simulink model "MARCH_v1_5_stairs"  (R2016a)
settings: Solver=FixedStepDiscrete  StartTime=0.0  StopTime=inf  FixedStep=0.001  RelTol=1e-3
InitFcn:
  | % Change dir to model location
  | cd(fileparts(which(bdroot)));
  | 
  | init_model
  | initialize_model_testingBlocks
StartFcn:
  | cd(fileparts(which(bdroot)));
StopFcn:
  | cd(fileparts(which(bdroot)));
model workspace (MAT data in the model file):
  localValue = 1
  targetValue = 0
undefined symbols (not defined in the file or in its folder): Hip_HAA, Left_Leg, Right_Leg
libraries: xpcethercatlib x71, slrtlib x7, simulink x1, aerolibanimutils x1, dspnetwork x1
(part 2 of 3)

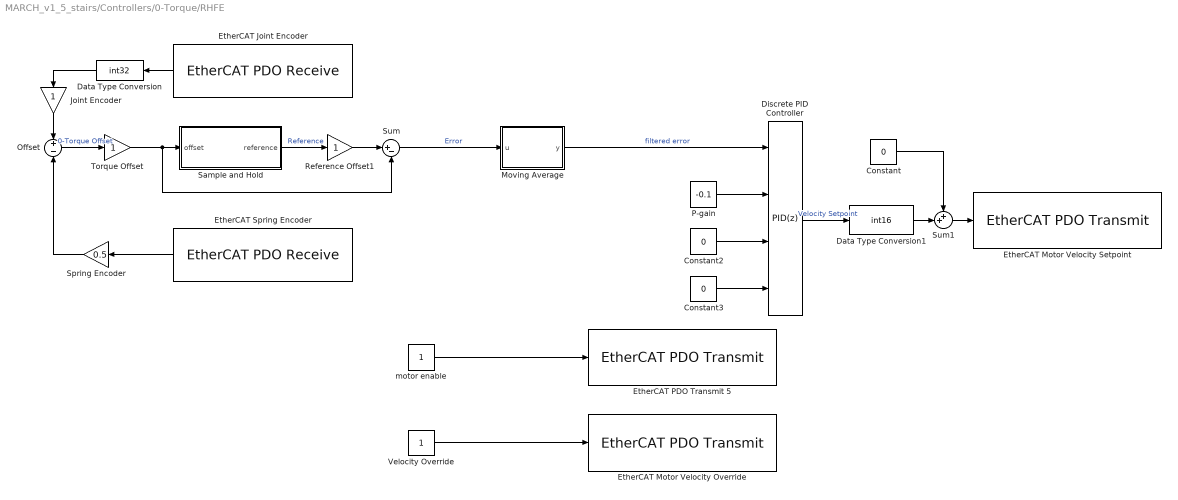
== system MARCH_v1_5_stairs/Controllers/0-Torque/RHFE ==
  Constant : Constant  Value=0  OutDataTypeStr=int16
  Constant2 : Constant  Value=0
  Constant3 : Constant  Value=0
  Data Type Conversion : DataTypeConversion  OutDataTypeStr=int32
  Data Type Conversion1 : DataTypeConversion  OutDataTypeStr=int16
  Discrete PID Controller : simulink/Continuous/PID Controller  Controller=PID  TimeDomain=Discrete-time  SampleTime=-1  IntegratorMethod=Forward Euler  FilterMethod=Forward Euler  Form=Parallel  UseFilter=off  ControllerParametersSource=external  P=-0.7  I=0  D=0  N=100  InitialConditionSource=internal  InitialConditionForIntegrator=0  InitialConditionForFilter=0  ExternalReset=none  LimitOutput=on  UpperSaturationLimit=500  LowerSaturationLimit=-500  LinearizeAsGain=off  AntiWindupMode=none  Kb=1  TrackingMode=off  Kt=1  PParamMin=[]  PParamMax=[]  IParamMin=[]  IParamMax=[]  DParamMin=[]  DParamMax=[]  NParamMin=[]  NParamMax=[]  KbParamMin=[]  KbParamMax=[]  KtParamMin=[]  KtParamMax=[]  POutMin=[]  POutMax=[]  IOutMin=[]  IOutMax=[]  DOutMin=[]  DOutMax=[]  NOutMin=[]  NOutMax=[]  KbOutMin=[]  KbOutMax=[]  KtOutMin=[]  KtOutMax=[]  IntegratorOutMin=[]  IntegratorOutMax=[]  FilterOutMin=[]  FilterOutMax=[]  SumOutMin=[]  SumOutMax=[]  SumOutDataTypeStr=int16  SumI1OutMin=[]  SumI1OutMax=[]  SumI2OutMin=[]  SumI2OutMax=[]  SumI3OutMin=[]  SumI3OutMax=[]  SumDOutMin=[]  SumDOutMax=[]  SaturationOutMin=[]  SaturationOutMax=[]  IntegratorContinuousStateAttributes=''  IntegratorStateMustResolveToSignalObject=off  IntegratorRTWStateStorageClass=Auto  FilterContinuousStateAttributes=''  FilterStateMustResolveToSignalObject=off  FilterRTWStateStorageClass=Auto  DifferentiatorICPrevScaledInput=0  DifferentiatorOutMin=[]  DifferentiatorOutMax=[]
  EtherCAT Joint Encoder : xpcethercatlib/EtherCAT PDO Receive  Priority=2  sig_name=Right_Leg.Inputs.H_jointAngle  sig_offset=1832  sig_type=uint32  type_size=32  sig_dim=1  device_id=0  sample_time=0.001000
  EtherCAT Motor Velocity Override : xpcethercatlib/EtherCAT PDO Transmit   Priority=3  sig_name=Right_Leg.Outputs.H_data[4]  sig_offset=2088  sig_type=int32  type_size=32  sig_dim=1  device_id=0  sample_time=0.001000
  EtherCAT Motor Velocity Setpoint : xpcethercatlib/EtherCAT PDO Transmit   Priority=3  sig_name=Right_Leg.Outputs.H_velocitySetPoint  sig_offset=1832  sig_type=int16  type_size=16  sig_dim=1  device_id=0  sample_time=0.001000
  EtherCAT PDO Transmit 5 : xpcethercatlib/EtherCAT PDO Transmit   Priority=3  sig_name=Right_Leg.Outputs.H_motorEnable  sig_offset=1880  sig_type=uint8  type_size=8  sig_dim=1  device_id=0  sample_time=0.001000
  EtherCAT Spring Encoder : xpcethercatlib/EtherCAT PDO Receive  Priority=2  sig_name=Right_Leg.Inputs.H_springAngle  sig_offset=1864  sig_type=uint32  type_size=32  sig_dim=1  device_id=0  sample_time=0.001000
  Joint Encoder : Gain  OutDataTypeStr=int32
  Moving Average : MATLAB Function  TreatAsAtomicUnit=on
  Offset : Sum  Inputs=+|-
  P-gain : Constant  Value=-0.1
  Reference Offset1 : Gain  OutDataTypeStr=int32
  Sample and Hold : MATLAB Function  TreatAsAtomicUnit=on
  Spring Encoder : Gain  Gain=0.5  OutDataTypeStr=int32
  Sum : Sum  Inputs=|+-  AccumDataTypeStr=uint32
  Sum1 : Sum  Inputs=++|
  Torque Offset : Gain  OutDataTypeStr=int32
  Velocity Override : Constant  OutDataTypeStr=int32
  motor enable : Constant  OutDataTypeStr=uint8
  wires:
  EtherCAT Joint Encoder/1 -> Data Type Conversion/1
  EtherCAT Spring Encoder/1 -> Spring Encoder/1
  Offset/1 -> Torque Offset/1  "0-Torque Offset"
  Sample and Hold/1(reference) -> Reference Offset1/1  "Reference"
  Sum/1 -> Moving Average/1(u)  "Error"
  Velocity Override/1 -> EtherCAT Motor Velocity Override/1
  Spring Encoder/1 -> Offset/2
  Data Type Conversion/1 -> Joint Encoder/1
  Joint Encoder/1 -> Offset/1
  Torque Offset/1 -> Sample and Hold/1(offset), Sum/2
  Reference Offset1/1 -> Sum/1
  Sum1/1 -> EtherCAT Motor Velocity Setpoint/1
  Discrete PID Controller/1 -> Data Type Conversion1/1  "Velocity Setpoint"
  Constant/1 -> Sum1/1
  motor enable/1 -> EtherCAT PDO Transmit 5/1
  Data Type Conversion1/1 -> Sum1/2
  P-gain/1 -> Discrete PID Controller/2
  Constant2/1 -> Discrete PID Controller/3
  Constant3/1 -> Discrete PID Controller/4
  Moving Average/1(y) -> Discrete PID Controller/1  "filtered error"

== system MARCH_v1_5_stairs/Controllers/Continuous Gait/Slider ==

== system MARCH_v1_5_stairs/Controllers/Hold/Motor enable ==
  MotorEnableFlag : Inport
  Demux : Demux  Outputs=6
  Enable LHAA : xpcethercatlib/EtherCAT PDO Transmit   Priority=3  sig_name=Hip_HAA.Outputs.L_motorEnable  sig_offset=256  sig_type=uint8  type_size=8  sig_dim=1  device_id=0  sample_time=0.001000
  Enable LHFE : xpcethercatlib/EtherCAT PDO Transmit   Priority=3  sig_name=Left_Leg.Outputs.H_motorEnable  sig_offset=1192  sig_type=uint8  type_size=8  sig_dim=1  device_id=0  sample_time=0.001000
  Enable LKFE : xpcethercatlib/EtherCAT PDO Transmit   Priority=3  sig_name=Left_Leg.Outputs.K_motorEnable  sig_offset=1480  sig_type=uint8  type_size=8  sig_dim=1  device_id=0  sample_time=0.001000
  Enable RHAA : xpcethercatlib/EtherCAT PDO Transmit   Priority=3  sig_name=Hip_HAA.Outputs.R_motorEnable  sig_offset=560  sig_type=uint8  type_size=8  sig_dim=1  device_id=0  sample_time=0.001000
  Enable RHFE : xpcethercatlib/EtherCAT PDO Transmit   Priority=3  sig_name=Right_Leg.Outputs.H_motorEnable  sig_offset=1880  sig_type=uint8  type_size=8  sig_dim=1  device_id=0  sample_time=0.001000
  Enable RKFE : xpcethercatlib/EtherCAT PDO Transmit   Priority=3  sig_name=Right_Leg.Outputs.K_motorEnable  sig_offset=2168  sig_type=uint8  type_size=8  sig_dim=1  device_id=0  sample_time=0.001000
  wires:
  Demux/3 -> Enable RKFE/1
  Demux/6 -> Enable LKFE/1
  Demux/5 -> Enable LHFE/1
  Demux/2 -> Enable RHFE/1
  MotorEnableFlag/1 -> Demux/1
  Demux/4 -> Enable LHAA/1
  Demux/1 -> Enable RHAA/1

== system MARCH_v1_5_stairs/EtherCAT Joint Setpoints/exoskeleton/EtherCAT Joint Communication ==
  Joint Setpoints : Inport
  Demux : Demux  Outputs=6
  "EtherCAT PDO Transmit " : xpcethercatlib/EtherCAT PDO Transmit   Priority=3  sig_name=Hip_HAA.Outputs.R_jointSetPoint  sig_offset=528  sig_type=uint32  type_size=32  sig_dim=1  device_id=0  sample_time=0.001000
  EtherCAT PDO Transmit 1 : xpcethercatlib/EtherCAT PDO Transmit   Priority=3  sig_name=Right_Leg.Outputs.H_jointSetPoint  sig_offset=1848  sig_type=uint32  type_size=32  sig_dim=1  device_id=0  sample_time=0.001000
  EtherCAT PDO Transmit 2 : xpcethercatlib/EtherCAT PDO Transmit   Priority=3  sig_name=Right_Leg.Outputs.K_jointSetPoint  sig_offset=2136  sig_type=uint32  type_size=32  sig_dim=1  device_id=0  sample_time=0.001000
  EtherCAT PDO Transmit 3 : xpcethercatlib/EtherCAT PDO Transmit   Priority=3  sig_name=Hip_HAA.Outputs.L_jointSetPoint  sig_offset=224  sig_type=uint32  type_size=32  sig_dim=1  device_id=0  sample_time=0.001000
  EtherCAT PDO Transmit 4 : xpcethercatlib/EtherCAT PDO Transmit   Priority=3  sig_name=Left_Leg.Outputs.H_jointSetPoint  sig_offset=1160  sig_type=uint32  type_size=32  sig_dim=1  device_id=0  sample_time=0.001000
  EtherCAT PDO Transmit 5 : xpcethercatlib/EtherCAT PDO Transmit   Priority=3  sig_name=Left_Leg.Outputs.K_jointSetPoint  sig_offset=1448  sig_type=uint32  type_size=32  sig_dim=1  device_id=0  sample_time=0.001000
  wires:
  Demux/5 -> EtherCAT PDO Transmit 4/1
  Demux/6 -> EtherCAT PDO Transmit 5/1
  Demux/4 -> EtherCAT PDO Transmit 3/1
  Demux/1 -> "EtherCAT PDO Transmit "/1
  Demux/2 -> EtherCAT PDO Transmit 1/1
  Joint Setpoints/1 -> Demux/1
  Demux/3 -> EtherCAT PDO Transmit 2/1

== system MARCH_v1_5_stairs/Input Device/Generate random block signal safety/Create peak1 ==
  In1 : Inport
  Delay : Delay  DelayLength=1
  Greater than 0 : MATLAB Function  TreatAsAtomicUnit=on
  Sum : Sum  Inputs=|-+
  Out1 : Outport
  wires:
  Sum/1 -> Greater than 0/1(peak)
  In1/1 -> Sum/2, Delay/1
  Delay/1 -> Sum/1
  Greater than 0/1(signal) -> Out1/1

== system MARCH_v1_5_stairs/Input Device/Generate random block signal safety/Create peak2 ==
  In1 : Inport
  Delay : Delay  DelayLength=1
  Greater than 0 : MATLAB Function  TreatAsAtomicUnit=on
  Sum : Sum  Inputs=|-+
  Out1 : Outport
  wires:
  Sum/1 -> Greater than 0/1(peak)
  In1/1 -> Sum/2, Delay/1
  Delay/1 -> Sum/1
  Greater than 0/1(signal) -> Out1/1

== system MARCH_v1_5_stairs/Input Device/Generate random block signal safety/Create peak3 ==
  In1 : Inport
  Delay : Delay  DelayLength=1
  Greater than 0 : MATLAB Function  TreatAsAtomicUnit=on
  Sum : Sum  Inputs=|-+
  Out1 : Outport
  wires:
  Sum/1 -> Greater than 0/1(peak)
  In1/1 -> Sum/2, Delay/1
  Delay/1 -> Sum/1
  Greater than 0/1(signal) -> Out1/1

== system MARCH_v1_5_stairs/Input Device/Generate random block signal trigger/Create peak1 ==
  In1 : Inport
  Delay : Delay  DelayLength=1
  Greater than 0 : MATLAB Function  TreatAsAtomicUnit=on
  Sum : Sum  Inputs=|-+
  Out1 : Outport
  wires:
  Sum/1 -> Greater than 0/1(peak)
  In1/1 -> Sum/2, Delay/1
  Delay/1 -> Sum/1
  Greater than 0/1(signal) -> Out1/1

== system MARCH_v1_5_stairs/Input Device/Generate random block signal trigger/Create peak2 ==
  In1 : Inport
  Delay : Delay  DelayLength=1
  Greater than 0 : MATLAB Function  TreatAsAtomicUnit=on
  Sum : Sum  Inputs=|-+
  Out1 : Outport
  wires:
  Sum/1 -> Greater than 0/1(peak)
  In1/1 -> Sum/2, Delay/1
  Delay/1 -> Sum/1
  Greater than 0/1(signal) -> Out1/1

== system MARCH_v1_5_stairs/Input Device/Generate random block signal trigger/Create peak3 ==
  In1 : Inport
  Delay : Delay  DelayLength=1
  Greater than 0 : MATLAB Function  TreatAsAtomicUnit=on
  Sum : Sum  Inputs=|-+
  Out1 : Outport
  wires:
  Sum/1 -> Greater than 0/1(peak)
  In1/1 -> Sum/2, Delay/1
  Delay/1 -> Sum/1
  Greater than 0/1(signal) -> Out1/1

== matlab function MARCH_v1_5_stairs/Reachability/MATLAB Function ==
  data: q input size=6; q_out output size=6; err output size=6
function [q_out, err] = fcn(q)

joint_limit_min = [-20 -109 -3 -23 -109 -3]'/180*pi;
joint_limit_max = [23 21 121 20 21 121]'/180*pi;

n = size(q,2);
%% Check if all joints are within limits

err = imag(q)~=0 | q<repmat(joint_limit_min,n,1) | q>repmat(joint_limit_max,n,1);
q_out = q;

== matlab function MARCH_v1_5_stairs/Controllers/Continuous Gait/Trajectory ==
  data: stepHeight input; q output; done output; stepLength input; q input size=[1 6]; torso_z output; debugIn input; base output; debug output
function [q,done, torso_z, base, debug]= fcn(stepHeight,stepLength,q,debugIn)
%#codegen

persistent r splineCtrl i trajectory fullStep fullWeightShift torsoTrajectory weightShiftRatio;

%% Initialize all variables
if(isempty(splineCtrl))
    splineCtrl = splineController();
end

if(isempty(fullStep))
    fullStep = 0;
    fullWeightShift = 0;
end

if(isempty(r))
    % Get frequency of the model
    r = robotics();
    r.base = 1;
    
end

if(isempty(i))
    i = 0;
end

if(isempty(trajectory))
    trajectory = [];
    torsoTrajectory = [];
end

if(isempty(weightShiftRatio))
    weightShiftRatio = 0;
end
%% Logic
% Only run this for the beginning of the swing
r.setTorsoHeight(debugIn);
if(~i)
    
    splineCtrl.method('circle');
    % We set the method of whether we want an analytically generated spline
    % or a spline directly from the database.
    % Options: 'circle' and 'stairs'
    splineCtrl.setStepLength(stepLength).setStepHeight(stepHeight);
    if(~fullStep)
        trajectory = splineCtrl.method('circle').setVelocity(0.7).getHalfStep();
        fullStep = 1;
    else
        trajectory = splineCtrl.method('circle').setVelocity(0.7).getFullStep();
    end
    
    % Transform the spline to the correct frame based on which foot is
    % swinging
    trajectory = r.transformSpline(trajectory);
    
    
    torso_delta = [0 0.0 0];
    
    % Weight shift to base foot
    if(r.base == 1)
        torso_delta(2) = abs(torso_delta(2));
    else
        torso_delta(2) = -abs(torso_delta(2));
    end
    
    if(~fullWeightShift)
        torsoTrajectory = splineCtrl.getHalfWeightShift(torso_delta);
        fullWeightShift = 1;
    else
        torsoTrajectory = splineCtrl.getFullWeightShift(torso_delta);
    end
    
    i = i+1;
end

r.point = [trajectory(1,i) trajectory(2,i) trajectory(3,i)];
debug = r.point;
% r.step(weightShiftRatio(i));
r.weightShift(torsoTrajectory(i,:));

r.inverseKinematics();
q = r.q;

torso_z = r.torso_z;

% Set final values as initial values for the next iteration
r.refresh();

% Reset iterator after we're done with the trajectory, otherwise we
% increment the counter and continue iterating as simulink continues
% sampling
if( i < (length(trajectory)))
    i = i+1;
    done = 0;
else
    i = 0;
    r.switchFoot(r.base);
    done = 1;
end

% Output which foot is currently ON THE GROUND
base = r.base;
end

== matlab function MARCH_v1_5_stairs/Controllers/Continuous Gait/Torso Trajectory ==
  data: desired input; current input; z output
function z = fcn(desired, current)
%#codegen

persistent trajectory i desiredPersistent;

% Speed at which we home in SAMPLES
samples = 1000;

if (isempty(i))
    i = 0;
    
    % Hack to fix initial condition of delay during init phase
    current = desired;
end

if(isempty(desiredPersistent))
    desiredPersistent = desired;
end

if(isempty(trajectory))
    trajectory = linspace(current,desiredPersistent,samples);
end

if(desiredPersistent ~= desired)
    trajectory = linspace(current,desired,samples);
    desiredPersistent = desired;
    i = 0;
end

if(i < samples)
    i = i+1;
end

z = trajectory(i);

== matlab function MARCH_v1_5_stairs/Controllers/Switcher ==
  data: index output; i input; enable output
function [index, enable]= fcn(i)
%#codegen

% This function is supposed to take a state and switch between controllers.
% Currently it directly routes the input argument as the index. In the
% future this can be something different so I have left it open for
% future modifications.

% The u vector represents the controllers. When the vector consists out of
% zeros it will not enable any controller. In the case that an index is set
% to a non zero value, the controller which belongs to that index will be
% enabled.
u = zeros(10,1);

u(i) = 2;

index = i;
enable = u;

== matlab function MARCH_v1_5_stairs/EtherCAT Joint Data In/MATLAB Function ==
  data: encoderValue input; angles output; par parameter
function angles = convertToJointAngles(encoderValue, par)
angles = zeros(6,1);

for i = 1:6
    angles(i) = enc2rad(encoderValue(i), i, par);
end

== matlab function MARCH_v1_5_stairs/Controllers/0-Torque/RHFE/Moving Average ==
  data: u input; y output
function y = fcn(u)

persistent array i;

if(isempty(array))
   array = zeros(1,100);
   i = 1;
end

if(i > 100)
   i = 1; 
end

array(i) = u;
i = i+1;
y = mean(array);

== matlab function MARCH_v1_5_stairs/Controllers/Walking/Trajectory ==
  data: base input; q output; done output; action input; stepType input; q input size=[1 6]; torsoHeight input; stepHeight input; stepLength input; stepVelocity input
function [q,done]= fcn(base,action,stepType, q, torsoHeight,stepHeight, stepLength, stepVelocity)
%#codegen

persistent r splineCtrl i triggerPersistent trajectory hold fullWeightShift timeCurve weightShiftRatio;

%% Initialize all variables
if(isempty(splineCtrl))
    splineCtrl = splineController();
end

if(isempty(fullWeightShift))
    fullWeightShift = 0;
end

% stepType can be 0,1 or 2. 0 = half step forward, 1 is full step, 2 is
% half step trailing
if(isempty(stepType))
    stepType = 0;
end

if(isempty(r))
    % Get frequency of the model
    r = robotics();
    r.base = base;
    timeCurve = [0 0 0];
end

if(isempty(hold))
    hold = 0;
end

if(isempty(i))
    i = 0;
end

if(isempty(triggerPersistent))
    triggerPersistent = action;
end


if(isempty(trajectory))
    trajectory = [0 0 0];
end

if(isempty(weightShiftRatio))
    weightShiftRatio = 0;
end
    
%% Logic
% Only run this for the beginning of the swing
done = 0;

% Reset values if trigger is toggled.
if(triggerPersistent ~= action)
    r.base = base;
    i = 0;
    hold = 0;
    triggerPersistent = action;
end

% Hold exoskeleton in same position after a single step
if(hold)
    q = r.q;
    done = 1;
    return
end

if(~i)
    % weightShiftRatio(end)
    % Foot Trajectory
    splineCtrl.method('circle');
    splineCtrl.setStepHeight(stepHeight).setStepLength(stepLength);
    if(~stepType || stepType == 2)
        trajectory = splineCtrl.method('circle').setVelocity(stepVelocity).getHalfStep();
    else
        trajectory = splineCtrl.method('circle').setVelocity(stepVelocity).getFullStep();
    end
    
    trajectory = r.transformSpline(trajectory);
    
    if(~stepType && r.base == 1)
        weightShiftRatio = linspace(0.5,0.7,length(trajectory));
    end
    
    if(~stepType && r.base == 3)
        weightShiftRatio = linspace(0.5,0.3,length(trajectory));
    end    
    
    % Get trajectory of torso based on the weight shift. WeightShiftRatio
    % is zero --> torso on right foot, WeightShiftRatio is 1 --> torso on
    % left foot
    if(stepType == 1 && r.base == 1)
        weightShiftRatio = linspace(0.3,0.7,length(trajectory));
    end
    
    if(stepType == 1 && r.base == 3)
        weightShiftRatio = linspace(0.7,0.3,length(trajectory));
    end
    
    % Get trajectory of torso based on the weight shift. WeightShiftRatio
    % is zero --> torso on right foot, WeightShiftRatio is 1 --> torso on
    % left foot
    if(stepType == 2 && r.base == 1)
        weightShiftRatio = linspace(0.3,0.5,length(trajectory));
    end
    
    if(stepType == 2 && r.base == 3)
        weightShiftRatio = linspace(0.7,0.5,length(trajectory));
    end

    timeCurve = splineCtrl.getEaseTimeCurve();
    
    i = i+1;
end
r.torso_z = torsoHeight;

r.point = [splineCtrl.easeTrajectory(trajectory(1,:),i,timeCurve) splineCtrl.easeTrajectory(trajectory(2,:),i,timeCurve) splineCtrl.easeTrajectory(trajectory(3,:),i,timeCurve)];
% r.step(); 
r.step(weightShiftRatio(i));
% r.weightShift(torsoTrajectory(i,:));
r.inverseKinematics();

q = r.q;
% torso(i,:) = r.torso;

% Set final values as initial values for the next iteration
r.refresh();

% Reset iterator after we're done with the trajectory, otherwise we
% increment the counter and continue iterating as simulink continues
% sampling
if( i < (length(trajectory)))
    i = i+1;
else
    hold = 1;
end

end

== matlab function MARCH_v1_5_stairs/Controllers/Hold/MATLAB Function ==
  data: q_in input size=[1 6]; action input; q_out output double size=[1 6]; reset input; motorEnable output
function [q_out, motorEnable] = fcn(q_in,action,reset)
persistent q_hold hold action_persistent

if(isempty(q_hold))
   q_hold = zeros(1,6); 
   hold = 0;
end

if (isempty(action_persistent))
    action_persistent = action;
end

if(reset)
   hold = 0; 
end

if (action_persistent ~= action)
    hold = 0;
    action_persistent = action;
end

if(~hold)
    q_hold = q_in;
    hold = 1;
end

motorEnable = uint8(zeros(1,6));

if (hold)
    motorEnable = uint8(ones(1,6));
end

q_out = q_hold;

== matlab function MARCH_v1_5_stairs/Input Device/Generate random block signal safety/Create peak1/Greater than 0 ==
  data: peak input; signal output
function signal  = fcn(peak)


if peak >= 0
    signal = peak;
else
    signal = 0;
    
    
end

== matlab function MARCH_v1_5_stairs/State Machine/Create peak3/Greater than 0 ==
  data: peak input; signal output
function signal  = fcn(peak)


if peak >= 0
    signal = peak;
else
    signal = 0;
    
    
end

== matlab function MARCH_v1_5_stairs/Controllers/Point & Go/Trajectory ==
  data: base input; q output; action input; point input; q input size=[1 6]; debugOut output; debugIn input
function [q,debugOut]= fcn(base,action, point,q,debugIn)
%#codegen

persistent r splineCtrl i triggerPersistent trajectory fullStep hold pointPersistent;

%% Initialize all variables
if(isempty(splineCtrl))
    splineCtrl = splineController();
end


if(isempty(fullStep))
    fullStep = 0;
end

if(isempty(r))
    r = robotics();
    r.base = base;
    
end

if(isempty(hold))
    hold = 0;
end

if(isempty(i))
    i = 0;
end

if(isempty(triggerPersistent))
    triggerPersistent = action;
end

if(isempty(pointPersistent))
    pointPersistent = point;
end

if(isempty(trajectory))
    trajectory = [0 0];
end

%% Logic

% Reset values if trigger is toggled.
if(triggerPersistent ~= action)
    r.base = base;
    i = 0;
    hold = 0;
    triggerPersistent = action;
end


% Hold exoskeleton in same position after a single step
if(hold)
    debugOut = r.torso_z;
    q = r.q;
    return
end

if(~i)
    
    % We set the method of whether we want an analytically generated spline
    % or a spline directly from the database.
    % Options: 'circle' and 'stairs'
    splineCtrl.setStepHeight(0.3);
    trajectory = splineCtrl.method('circle').getStepFromPoint(point);
    
    
    
    % Transform the spline to the correct frame based on which foot is
    % swinging
    trajectory = r.transformSpline(trajectory);
    
    i = i+1;
end

r.point = [trajectory(1,i) trajectory(2,i) trajectory(3,i)];

r.stepPosture();
r.inverseKinematics();

q = r.q;
debugOut = r.torso_z;

% Set final values as initial values for the next iteration
r.refresh();

% Reset iterator after we're done with the trajectory, otherwise we
% increment the counter and continue iterating as simulink continues
% sampling
if( i < (length(trajectory)))
    i = i+1;
else
    hold = 1;
end

end

== matlab function MARCH_v1_5_stairs/State Machine/Input Interpreter Safety ==
  data: rightIn input; rightOut output; leftIn input; leftOut output; bothOut output
function [rightOut, leftOut, bothOut]= fcn(rightIn, leftIn)

persistent countRight countLeft countBoth

if (isempty(countRight)||isempty(countLeft)||isempty(countBoth));
    countRight = 0;
    countLeft = 0;
    countBoth = 0;
    rightOut = 0;
    leftOut = 0;
    bothOut = 0;
end

threshold = 700;


if (rightIn == 0 && leftIn == 0)
    rightOut = 0;
    leftOut = 0;
    bothOut = 0;
    countRight = 0;
    countLeft = 0;
    countBoth = 0;
elseif (rightIn == 1 && leftIn ~= 1)
    countRight = countRight + 1;
    countLeft = 0;
    countBoth = 0;
    if countRight == threshold
        rightOut = 1;
        leftOut = 0;
        bothOut = 0;
        countRight = 0;
    else
        rightOut = 0;
        leftOut = 0;
        bothOut = 0;
    end
elseif (leftIn == 1 && rightIn ~= 1)
    countRight = 0;
    countLeft = countLeft + 1;
    countBoth = 0;
    if countLeft == threshold
        rightOut = 0;
        leftOut = 1;
        bothOut = 0;
        countLeft = 0;
    else
        rightOut = 0;
        leftOut = 0;
        bothOut = 0;
    end
elseif (rightIn == 1 && leftIn == 1)
    countRight = 0;
    countLeft = 0;
    countBoth = countBoth + 1;
    if countBoth == threshold
        rightOut = 0;
        leftOut = 0;
        bothOut = 1;
    else
        rightOut = 0;
        leftOut = 0;
        bothOut = 0;
    end
else
    rightOut = -1;
    leftOut = -1;
    bothOut = -1;
end

== matlab function MARCH_v1_5_stairs/EtherCAT Joint Setpoints/exoskeleton/MATLAB Function ==
  data: jointAngle input; encVal output; par parameter
function encVal = convertToEncoderValues(jointAngle, par)
encVal = zeros(6,1);

for i = 1:6
    encVal(i) = rad2enc(jointAngle(i), i, par);
end

== matlab function MARCH_v1_5_stairs/Controllers/StandUp/Trajectory ==
  data: done output; q output; action input; q_i input size=[1 6]; debugIn input
function [done,q] = fcn(action,q_i,debugIn)
%#codegen

persistent r splineCtrl i q_t n hipDelay;

%% Initialize all variables
if(isempty(splineCtrl))
    splineCtrl = splineController();
end

if(isempty(r))
    % Get frequency of the model
    r = robotics();
    
end

if(isempty(q_t))
    q_t = [0 0 0 0 0 0];
    hipDelay = [0 0];
end

if(isempty(i))
    i = 0;
    n = 0;
end


%% Logic
done = 0;

% Prepare for standup by moving the hip forward
if(n == 0 && i == 0)
    q_f = [0 -1.9 q_i(3) 0 -1.9 q_i(6)];
    splineCtrl.samples = 1500;
    q_t = splineCtrl.getJointTrajectory(q_i,q_f);
   
    i = i+1;
end

% Run startup procedure
if(n == 1 && i == 0)
    % Calculate final position based on robotics parameters
    r.setTorsoHeight(debugIn);
    r.refresh();
    r.inverseKinematics();
    q_f = r.q;
    
    splineCtrl.samples = 3000;
    q_t = splineCtrl.getJointTrajectory(q_i,q_f);

    % The hip rotation will play back halfway through the samples
    hipDelay = splineCtrl.getCustomEaseTimeCurve(0.3,1);
    
    i = i+1;
    %q_t = splineCtrl.ease(q_t);
end

q = q_t(i,:);

% Slow down the hip trajectory only when standing up
if(n == 1)
    q(2) = splineCtrl.easeTrajectory(q_t(:,2),i,hipDelay);
    q(5) = splineCtrl.easeTrajectory(q_t(:,5),i,hipDelay);
end

if(i < length(q_t))
    i = i+1;
else
    if(n == 0)
        % Reset iterator
        i = 0;
        n = 1;
    else
        done = 1;
    end
end

end

== matlab function MARCH_v1_5_stairs/State Machine/Input Interpreter Triggers ==
  data: rightIn input; rightOut output; leftIn input; leftOut output; bothOut output
function [rightOut, leftOut, bothOut]= fcn(rightIn, leftIn)

persistent countRight countLeft countBoth

if (isempty(countRight)||isempty(countLeft)||isempty(countBoth));
    countRight = 0;
    countLeft = 0;
    countBoth = 0;
    rightOut = 0;
    leftOut = 0;
    bothOut = 0;
end

threshold = 700;


if (rightIn == 0 && leftIn == 0)
    rightOut = 0;
    leftOut = 0;
    bothOut = 0;
    countRight = 0;
    countLeft = 0;
    countBoth = 0;
elseif (rightIn == 1 && leftIn ~= 1)
    countRight = countRight + 1;
    countLeft = 0;
    countBoth = 0;
    if countRight == threshold
        rightOut = 1;
        leftOut = 0;
        bothOut = 0;
        countRight = 0;
    else
        rightOut = 0;
        leftOut = 0;
        bothOut = 0;
    end
elseif (leftIn == 1 && rightIn ~= 1)
    countRight = 0;
    countLeft = countLeft + 1;
    countBoth = 0;
    if countLeft == threshold
        rightOut = 0;
        leftOut = 1;
        bothOut = 0;
        countLeft = 0;
    else
        rightOut = 0;
        leftOut = 0;
        bothOut = 0;
    end
elseif (rightIn == 1 && leftIn == 1)
    countRight = 0;
    countLeft = 0;
    countBoth = countBoth + 1;
    if countBoth == threshold
        rightOut = 0;
        leftOut = 0;
        bothOut = 1;
    else
        rightOut = 0;
        leftOut = 0;
        bothOut = 0;
    end
else
    rightOut = -1;
    leftOut = -1;
    bothOut = -1;
end

== matlab function MARCH_v1_5_stairs/Controllers/Stairs/Torso Trajectory ==
  data: desired input; torsoTrajectory output size=[1 3]
function torsoTrajectory = fcn(desired)
%#codegen

persistent trajectory i desiredPersistent;

% Speed at which we home in SAMPLES
samples = 1000;

if (isempty(i))
    i = 0;
end

if(isempty(desiredPersistent))
    desiredPersistent = desired;
end

if(isempty(trajectory))   
    desiredPersistent = desired;
    
    trajectory = [linspace(0,desiredPersistent(1),samples)
        linspace(0,desiredPersistent(2),samples)
        linspace(0,desiredPersistent(3),samples) ]';
end

if(~isequal(desiredPersistent,desired))
    trajectory = [linspace(0,desired(1),samples)
        linspace(0,desired(2),samples)
        linspace(0,desired(3),samples) ]';
    
    desiredPersistent = desired;
    i = 0;
end

if(i < samples)
    i = i+1;
end

torsoTrajectory = trajectory(i,:);

== matlab function MARCH_v1_5_stairs/Controllers/Stairs/Trajectory ==
  data: base input; q output; action input; q input size=[1 6]; stepVelocity input; stepLength input; stairHeight input; seq input; done output
function [q,done] = fcn(base,action,q,stepVelocity,stepLength,stairHeight,seq)
%#codegen

persistent r s i j k l m hold trajectory weightShiftRatio timeCurve splineCtrl triggerPersistent;

%% Initialize all variables
if(isempty(splineCtrl))
    splineCtrl = splineController();
end

if(isempty(r))
    % Get frequency of the model
    r = robotics();
    r.base = base;
end

if(isempty(i) || isempty(j) || isempty(k) || isempty(l))
    i = 0;
    j = 0;
    k = 0;
    l = 0;
    m = 0;
end

if(isempty(trajectory))
    trajectory = [0 0 0];
end

if(isempty(triggerPersistent))
    triggerPersistent = action;
end

if(isempty(weightShiftRatio))
    weightShiftRatio = 0;
end

if(isempty(timeCurve))
    timeCurve = 0;
end

if(isempty(hold))
    hold = 0;
end

%% Logic
done = 0;

% Reset values if trigger is toggled.
if(triggerPersistent ~= action)
    r.base = base;
    i = 0;
    hold = 0;
    triggerPersistent = action;
end

% Hold exoskeleton in same position after a single step
if(hold)
    q = r.q;
    done = 1;
    return
end

% Initialisation of number of samples by use of the step Length and the
% step Velocity
splineCtrl.setStepLength(stepLength).setVelocity(stepVelocity).setStairHeight(stairHeight);
%% Weight shifting sequence
% This sequence will weight shift to the base leg. The entire sequence is
% wrapped inside an if statement to prevent this from executing after it
% has been completed. It is either this or a separate function block which
% would be a disaster because the classes are separate instances.


if(seq == 1)
    if (~i)
        r.torso_z = 0.9499;
        r.refresh(); % make sure initial position of torso has same heighit as set above
        
       % I tried to make a smooth weightShift using easeTrajectory but was
       % unsuccessfull, this is far out the fastest and easist solution.
        weightShiftRatio = splineCtrl.getWeightShiftRatioSpacing(0.5, 0.3);  
        
        i = i + 1;      
    end
    
    % Playback trajectory and return preventing doing the rest
    if(i < length(weightShiftRatio))
        r.weightShift(weightShiftRatio(i));
        r.inverseKinematics();
        q = r.q;
        i = i + 1;
    else
        q = r.q;
        
        % Init and enable step sequence
        r.refresh();
        j = 0; 
        done = 1;
        hold = 1;
    end
end

%% Step Sequence
% This sequence will step onto the stair
if(seq == 2)
    if(~j)
        r.base = base;
        % Generate the trajectory based on specific velocity (in m/s) for putting
        % the first leg on the stairs step
        trajectory = splineCtrl.method('stairs_lift').setStepLength(stepLength).setVelocity(stepVelocity).setStepHeightStairs().getStairStep();
        
        % Transform spline to location of foot
        trajectory = r.transformSpline(trajectory);
        
        % Perform the weightShift
        weightShiftRatio = linspace(weightShiftRatio(end),weightShiftRatio(end),length(trajectory));
        timeCurve = splineCtrl.getEaseTimeCurve();
        j = j + 1;
    end
    
    r.point = [splineCtrl.easeTrajectory(trajectory(1,:),j,timeCurve) splineCtrl.easeTrajectory(trajectory(2,:),j,timeCurve) splineCtrl.easeTrajectory(trajectory(3,:),j,timeCurve)];
    r.step(weightShiftRatio(j));
    r.inverseKinematics();
    q = r.q;

    r.refresh();
    
    if(j < length(trajectory))
        j = j+1;
    else
        j = 0;
        q = r.q;
        hold = 1;
        done = 1;
    end
    
end

%% Weightshift on stairs
% This sequence will make the weight be shifted on the leg on the stair
if(seq == 3)
    if(~k)
        r.base = base;
        % I tried to make a smooth weightShift using easeTrajectory but was
        % unsuccessfull, this is far out the fastest and easist solution.
        weightShiftRatio = splineCtrl.getWeightShiftRatioSpacing(weightShiftRatio(end), 0.7);
        
        k = k + 1;
    end
    
    % Playback trajectory and return preventing doing the rest
   
    r.weightShift(weightShiftRatio(k));
    r.inverseKinematics();
    q = r.q;
    
    r.refresh();
 
    if(k < length(weightShiftRatio))
        k = k + 1;
    else
        k = 0;
        q = r.q;
        
        % Init and enable step sequence
        r.refresh();
        k = 0;
        done = 1;
        hold = 1;
    end
end

%% Lifting the trailing leg
% This sequence will left the other leg on the stairs
if(seq == 4)
    if(~l)
        r.base = base;
        % Generate the trajectory based on specific velocity (in m/s) for putting
        % the first leg on the stairs step
        trajectory = splineCtrl.setStepLength(stepLength).setVelocity(stepVelocity).setStepHeightStairs().getTrailingStairStep();
        
        % Transform spline to location of foot
        trajectory = r.transformSpline(trajectory);
        
        weightShiftRatio = linspace(weightShiftRatio(end),weightShiftRatio(end),length(trajectory));
        
        timeCurve = splineCtrl.getEaseTimeCurve();
        
        l = l + 1;
    end 
    
    r.point = [splineCtrl.easeTrajectory(trajectory(1,:),l,timeCurve) splineCtrl.easeTrajectory(trajectory(2,:),l,timeCurve) splineCtrl.easeTrajectory(trajectory(3,:),l,timeCurve)];
    r.step(weightShiftRatio(l));
    r.inverseKinematics();
    q = r.q;

    r.refresh();
    
    if(l < length(trajectory))
        l = l+1;
    else
        l = 0;
        q = r.q;
        hold = 1;
        done = 1;
    end
    
end

%% Making the weightShift back to the middle
% This sequence shifts the MARCH back to the starting position
if(seq == 5)
    if(~m) 
        r.base = base;
        
        % I tried to make a smooth weightShift using easeTrajectory but was
        % unsuccessfull, this is far out the fastest and easist solution.
        weightShiftRatio = splineCtrl.getWeightShiftRatioSpacing(weightShiftRatio(end), 0.5); 
        
        m = m + 1;
    end
        
    r.weightShift(weightShiftRatio(m));
    r.inverseKinematics();
    q = r.q;
   
    r.refresh();
 
    if(m < length(weightShiftRatio))
        m = m + 1;
    else
        m = 0;
        q = r.q;
        
        % Init and enable step sequence
        r.refresh();
        m = 0;
        done = 1;
        hold = 1;
    end
end

weightShiftRatio(end)
end

== matlab function MARCH_v1_5_stairs/Controllers/0-Torque/RHFE/Sample and Hold ==
  data: offset input; reference output
function reference = fcn(offset)
%#codegen

persistent offsetPersistent hold;

if(isempty(offsetPersistent))
    offsetPersistent = int32(0);
    hold = 0;
end

if(offset > 0 && hold == 0)
    
    offsetPersistent = offset;
    hold = 1;
end

reference = offsetPersistent;

== stateflow chart MARCH_v1_5_stairs/State Machine/State Machine ==
  state InputDeviceCheck [commented out]
    en: controllerIndex = 1;
    en: action = 0;
    en: base = 0;
    en: stepType = 0;
    en: state = 0;
    state checkScrollClick [commented out]
      en: inpDevWorking = 0;
    state checkBothSafety [commented out]
      en: inpDevWorking = 0;
    state checkbothTrigger [commented out]
      en: inpDevWorking = 0;
    state InpDev [commented out]
      en: inpDevWorking = 1;
    (default) -> checkScrollClick [commented out] : [rightScrollMode == 1]
    checkScrollClick -> checkBothSafety [commented out] : [rightScrollClick == 1]
    checkBothSafety -> checkbothTrigger [commented out] : [bothSafety == 1]
    checkbothTrigger -> InpDev [commented out] : [bothTriggers == 1]
  state ZeroTorque
    en: controllerIndex = 1;
    en: action = 0;
    en: base = 0;
    en: stepType = 0;
    en: state = 1;
  state testingBypass
    en: controllerIndex = 1;
    en: action = 0;
    en: base = 0;
    en: stepType = 0;
    en: state = 9;
  state SitDown
    en: controllerIndex = 4;
    en: action = 0;
    en: base = 0;
    en: stepType = 0;
    en: state = 4;
  state HoldPosition
    en: controllerIndex = 2;
    en: action = 0;
    en: base = 0;
    en: stepType = 0;
    en: state = 2;
  state StandUp
    en: controllerIndex = 3;
    en: action = 0;
    en: base = 0;
    en: stepType = 0;
    en: state = 3;
  state HoldPosition1
    en: controllerIndex = 2;
    en: action = 0;
    en: base = 0;
    en: stepType = 0;
    en: state = 2;
  state DiscreteGait
    en: controllerIndex = 5;
    state standbyModeDiscr
      en: action = actionLocal;
      en: base = baseLocal;
      en: stepType = 0;
      en: state = 61;
      % satandby mode from discrete gait
      % exoskeleton finishes full step, makes complementary halfstep, then stands still
    state makeLeftHalfStepDiscr
      en: action = action+1;
      en: base = 1;
      en: stepType = 2;
      en: state = 61;
      baseLocal = base;
      actionLocal = action;
    state makeRightHalfStepDiscr
      en: action = action+1;
      en: base = 3;
      en: stepType = 2;
      en: state = 61;
      baseLocal = base;
      actionLocal = action;
    state startLeftHalfStepDiscr
      en: action = 1;
      en: base = 1;
      en: stepType = 0;
      en: state = 6;
      baseLocal = base
    state finishRightFullStepDiscr
      en: action = actionLocal;
      en: base = 3;
      en: stepType = 1;
      en: state = 61;
      baseLocal = base;
      % exoskeleton finishes right full step
    state finishLeftFullStepDiscr
      en: action = actionLocal;
      en: base = 1;
      en: stepType = 1;
      en: state = 61;
      baseLocal = base;
      % exoskeleton finishes left full step
    state makeLeftHalfStepDiscr1
      en: action = action+1;
      en: base = 1;
      en: stepType = 0;
      en: state = 62;
      baseLocal = base;
      actionLocal = action;
    state makeRightHalfStepDiscr3
      en: action = action+1;
      en: base = 3;
      en: stepType = 0;
      en: state = 62;
      baseLocal = base;
      actionLocal = action;
    state leftFullStepDiscr
      en: action = action+1;
      en: base = 1;
      en: stepType = 1;
      en: state = 6;
      baseLocal = base;
      actionLocal = action;
    state rightFullStepDiscr
      en: action = action+1;
      en: base = 3;
      en: stepType = 1;
      en: state = 6;
      baseLocal = base;
      actionLocal = action;
    state safeDiscr2Walk1
      en: action = actionLocal;
      en: base = baseLocal;
      en: stepType = 1;
      en: state = 62;
    state safeDiscr2Walk
      en: action = actionLocal;
      en: base = baseLocal;
      en: stepType = 1;
      en: state = 62;
    state safeModeDiscr
      en: action = actionLocal;
      en: base = baseLocal;
      en: stepType = 1;
      en: state = 62;
      % safemode from discr. gait
      % exoskeleton finishes full step, then stands still
    makeRightHalfStepDiscr3 -> standbyModeDiscr : [done == 1]
    makeLeftHalfStepDiscr1 -> standbyModeDiscr : [done == 1]
    standbyModeDiscr -> startLeftHalfStepDiscr [order 2] : [bothTriggers == 1]
    makeLeftHalfStepDiscr -> standbyModeDiscr : [done == 1]
    makeRightHalfStepDiscr -> standbyModeDiscr : [done == 1]
    finishLeftFullStepDiscr -> makeRightHalfStepDiscr : [done == 1]
    finishRightFullStepDiscr -> makeLeftHalfStepDiscr : [done == 1]
    startLeftHalfStepDiscr -> rightFullStepDiscr : [done == 1 && rightTrigger == 1]
    leftFullStepDiscr -> finishLeftFullStepDiscr [order 1] : [bothTriggers == 1]
    rightFullStepDiscr -> finishRightFullStepDiscr [order 1] : [bothTriggers == 1]
    (junction 178) -> makeRightHalfStepDiscr3 [order 2] : [baseLocal == 1]
    (junction 178) -> makeLeftHalfStepDiscr1 [order 1] : [baseLocal == 3]
    rightFullStepDiscr -> leftFullStepDiscr [order 2] : [done == 1 && leftTrigger ==  1]
    leftFullStepDiscr -> rightFullStepDiscr [order 2] : [done == 1 && rightTrigger == 1]
    safeDiscr2Walk1 -> leftFullStepDiscr [order 2] : [leftTrigger == 1 && baseLocal == 3]
    leftFullStepDiscr -> safeModeDiscr [order 3] : [bothSafety == 1]
    rightFullStepDiscr -> safeModeDiscr [order 3] : [bothSafety == 1]
    safeDiscr2Walk1 -> rightFullStepDiscr [order 1] : [rightTrigger == 1 && baseLocal == 1]
    safeDiscr2Walk -> safeDiscr2Walk1 : [done == 1]
    safeModeDiscr -> safeDiscr2Walk [order 1] : [bothSafety == 1]
    safeModeDiscr -> (junction 178) [order 2] : [bothTriggers == 1 && done == 1]
  state ContinuousGait
    en: controllerIndex = 5;
    state standbyModeCont
      en: action = actionLocal;
      en: base = baseLocal;
      en: stepType = 0;
      en: state = 51;
      % satandby mode from continuous gait
      % exoskeleton finishes full step, makes complementary halfstep, then stands still
    state makeLeftHalfStepCont
      en: action = action+1
      en: base = 1;
      en: stepType = 0;
      en: state = 51;
      baseLocal = base;
    state makeRightHalfStepCont
      en: action = action+1;
      en: base = 3;
      en: stepType = 0;
      en: state = 51;
      baseLocal = base;
      actionLocal = action;
    state startLeftHalfStepCont
      en: action = 1;
      en: base = 1;
      en: stepType = 0;
      en: state = 5;
      baseLocal = base
    state finishLeftFullStepCont
      en: action = actionLocal;
      en: base = 1;
      en: stepType = 1;
      en: state = 51;
      baseLocal = base;
      % exoskeleton finishes left full step
    state finishRightFullStepCont
      en: action = actionLocal
      en: base = 3;
      en: stepType = 1;
      en: state = 51;
      baseLocal = base;
      % exoskeleton finishes right full step
    state makeRightHalfStepCont1
      en: action = action+1;
      en: base = 3;
      en: stepType = 0;
      en: state = 52;
      baseLocal = base;
      actionLocal = action;
    state makeLeftHalfStepCont1
      en: action = action+1;
      en: base = 1;
      en: stepType = 0;
      en: state = 52;
      baseLocal = base;
      actionLocal = action
    state leftFullStepCont
      en: action = action+1;
      en: base = 1;
      en: stepType = 1;
      en: state = 5;
      baseLocal = base;
      actionLocal = action;
    state rightFullStepCont
      en: action = action+1
      en: base = 3;
      en: stepType = 1;
      en: state = 5;
      baseLocal = base;
      actionLocal = action;
    state safeCont2Walk
      en: action = actionLocal;
      en: base = baseLocal;
      en: stepType = 1;
      en: state = 52;
    state safeModeCont
      en: action = actionLocal;
      en: base = baseLocal;
      en: stepType = 1;
      en: state = 52;
      % safemode from cont. gait
      % exoskeleton finishes full step, then stands still
    makeRightHalfStepCont1 -> standbyModeCont : [done == 1]
    standbyModeCont -> startLeftHalfStepCont [order 2] : [bothTriggers == 1]
    makeLeftHalfStepCont1 -> standbyModeCont : [done == 1]
    makeRightHalfStepCont -> standbyModeCont : [done == 1]
    makeLeftHalfStepCont -> standbyModeCont : [done == 1]
    finishLeftFullStepCont -> makeRightHalfStepCont : [done == 1]
    finishRightFullStepCont -> makeLeftHalfStepCont : [done == 1]
    startLeftHalfStepCont -> rightFullStepCont : [done == 1]
    leftFullStepCont -> finishLeftFullStepCont [order 2] : [bothTriggers == 1]
    rightFullStepCont -> finishRightFullStepCont [order 1] : [bothTriggers == 1]
    (junction 172) -> makeRightHalfStepCont1 [order 2] : [baseLocal == 1]
    (junction 172) -> makeLeftHalfStepCont1 [order 1] : [baseLocal == 3]
    leftFullStepCont -> rightFullStepCont [order 3] : [done == 1]
    rightFullStepCont -> leftFullStepCont [order 3] : [done == 1]
    safeCont2Walk -> rightFullStepCont [order 1] : [done == 1 && baseLocal == 1]
    rightFullStepCont -> safeModeCont [order 2] : [bothSafety == 1]
    leftFullStepCont -> safeModeCont [order 1] : [bothSafety == 1]
    safeCont2Walk -> leftFullStepCont [order 2] : [done == 1 && baseLocal == 3]
    safeModeCont -> safeCont2Walk [order 1] : [bothSafety == 1]
    safeModeCont -> (junction 172) [order 2] : [bothTriggers == 1 && done == 1]
  state StairsWalking
    en: controllerIndex = 8;
    state initialWeightShift
      entry: action = 1;
      en: seq = 1;
      en: base = 1;
    state weightShiftStartingPosition
      en: action = action + 1;
      en: seq = 5;
      en: base = 1;
    state firstStepStairsLeftLeg
      en: action = action + 1;
      en: seq = 2;
      en: base = 1;
    state liftLegStairs
      en: action = action + 1;
      en: seq = 4;
      en: base = 3;
    state weightShiftStair
      en: action = action + 1;
      en: seq = 3;
      en: base = 3;
    initialWeightShift -> firstStepStairsLeftLeg : [done == 1]
    weightShiftStartingPosition -> initialWeightShift [order 1] : [done == 1 && rightScrollClick == 1]
    firstStepStairsLeftLeg -> weightShiftStair : [done == 1]
    liftLegStairs -> weightShiftStartingPosition : [done == 1]
    weightShiftStair -> liftLegStairs : [done == 1]
  (default) -> InputDeviceCheck [commented out] : [rightScrollMode == 0]
  checkScrollClick -> testingBypass [commented out] : [rightScrollMode == 9]
  (default) -> ZeroTorque
  ZeroTorque -> HoldPosition [order 1] : [rightScrollMode == 3 && rightScrollClick == 1]
  SitDown -> ZeroTorque [order 1] : [rightScrollMode == 1 && rightScrollClick == 1 && done == 1]
  HoldPosition -> ZeroTorque [order 1] : [rightScrollMode == 1 && rightScrollClick == 1]
  ZeroTorque -> startLeftHalfStepCont [order 3] : [rightScrollMode == 11]
  ZeroTorque -> initialWeightShift [order 2] : [rightScrollMode == 12]
  testingBypass -> HoldPosition : [rightScrollClick == 1]
  HoldPosition1 -> SitDown [order 1] : [rightScrollMode ==4 && rightScrollClick == 1]
  SitDown -> StandUp [order 2] : [rightScrollMode == 3 && rightScrollClick == 1 && done == 1]
  HoldPosition -> StandUp [order 2] : [rightScrollMode == 3 && bothTriggers == 1]
  StandUp -> HoldPosition1 : [done == 1]
  standbyModeCont -> HoldPosition1 [order 1] : [rightScrollMode == 3 && rightScrollClick == 1]
  standbyModeDiscr -> HoldPosition1 [order 1] : [rightScrollMode == 3 && rightScrollClick == 1]
  weightShiftStartingPosition -> HoldPosition1 [order 2] : [rightScrollMode == 3 && rightScrollClick == 1]
  HoldPosition1 -> startLeftHalfStepCont [order 2] : [rightScrollMode == 5 && rightScrollClick == 1]
  HoldPosition1 -> startLeftHalfStepDiscr [order 3] : [rightScrollMode == 6 && rightScrollClick == 1]
  weightShiftStartingPosition -> startLeftHalfStepDiscr [order 3] : [done ==1 && rightScrollMode == 13]
  data: rightTrigger input; leftTrigger input; bothTriggers input; rightSafety input; leftSafety input; bothSafety input; rightScrollMode input; rightScrollClick input; controllerIndex output; action output; base output; inpDevWorking local; done input; stepType output; state output; baseLocal local; actionLocal local; seq output

== matlab function MARCH_v1_5_stairs/Input Device/Generate random block signal safety/Create peak2/Greater than 0 ==
  data: peak input; signal output
function signal  = fcn(peak)


if peak >= 0
    signal = peak;
else
    signal = 0;
    
    
end

== matlab function MARCH_v1_5_stairs/Input Device/Generate random block signal safety/Create peak3/Greater than 0 ==
  data: peak input; signal output
function signal  = fcn(peak)


if peak >= 0
    signal = peak;
else
    signal = 0;
    
    
end

== matlab function MARCH_v1_5_stairs/Input Device/Generate random block signal safety/Rand. Block Func. Gen.1 ==
  data: u input; delayDurationInp input; blockDurationInp input; output output
function output  = fcn(u, delayDurationInp, blockDurationInp)

%% initialize the variable
persistent delayDuration blockDuration

if(isempty(blockDuration)||isempty(delayDuration))
    blockDuration = 0;
    delayDuration = 0;
    output = 0;
end

%% check if the delay and the block are done

doneDelay = (delayDuration <= 0);
doneBlock = (blockDuration <= 0);
done = (doneDelay && doneBlock);



%% Create delay and Block

if (u == 0 && done)
    output = 0;
elseif u == 1
    delayDuration = floor(1000*delayDurationInp);
    output = 0;
elseif not(doneDelay)
    delayDuration = delayDuration - 1;
    output = 0;
    if delayDuration == 0
        blockDuration = floor(1000*blockDurationInp);
        output = 1;
    end
elseif not(doneBlock)
    blockDuration = blockDuration - 1;
    output = 1;
else
    output = -1;
end


end

== matlab function MARCH_v1_5_stairs/Input Device/Generate random block signal safety/Rand. Block Func. Gen.4 ==
  data: delayDurationInp input; blockDurationInp input; u input; output output
function output  = fcn(delayDurationInp, blockDurationInp, u)

%% initialize the variable
persistent delayDuration blockDuration

if(isempty(blockDuration)||isempty(delayDuration))
    blockDuration = 0;
    delayDuration = 0;
    output = 0;
end



%% check if the delay and the block are done

doneDelay = (delayDuration <= 0);
doneBlock = (blockDuration <= 0);
done = (doneDelay && doneBlock);



%% Create delay and Block

if (u == 0 && done)
    output = 0;
elseif u == 1
    delayDuration = floor(1000*delayDurationInp);
    output = 0;
elseif not(doneDelay)
    delayDuration = delayDuration - 1;
    output = 0;
    if delayDuration == 0
        blockDuration = floor(1000*blockDurationInp);
        output = 1;
    end
elseif not(doneBlock)
    blockDuration = blockDuration - 1;
    output = 1;
else
    output = -1;
end


end

== matlab function MARCH_v1_5_stairs/Input Device/Generate random block signal safety/Saturation 2 ==
  data: u input; y output
function y = fcn(u)

min = 0.5;
max = 1.2;

if u <= min
    y = min;
elseif u >= max;
    y = max;
else
    y = u;
end

== matlab function MARCH_v1_5_stairs/Input Device/Generate random block signal safety/Saturation1 ==
  data: u input; y output
function y = fcn(u)

min = 0.1;
max = 0.3;

if u <= min
    y = min;
elseif u >= max;
    y = max;
else
    y = u;
end
